simulink model "TRANSMISION_MULTIPLEXADA60EB2"  (R2016a)
settings: Solver=VariableStepAuto  StartTime=0.0  StopTime=420800  RelTol=1e-3
libraries: commutil2 x14, commdigbbndpm3 x14, commsrccod2 x6, commchan3 x2, commsink2 x1
settings Model: Creator=Glynis  LastModifiedBy=Glynis

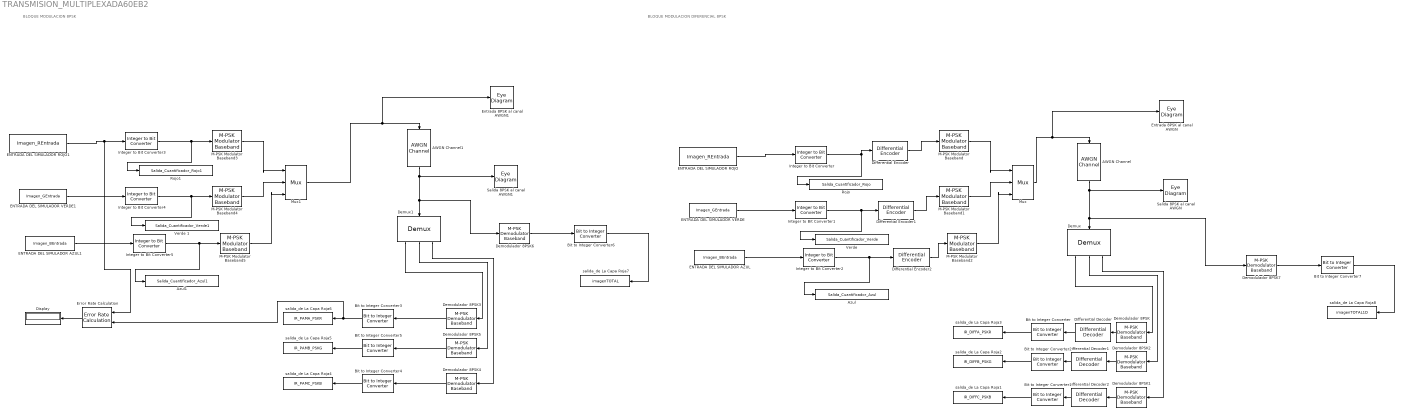
== system TRANSMISION_MULTIPLEXADA60EB2 ==
  note: BLOQUE MODULACION DIFERENCIAL 8PSK
  note: BLOQUE MODULACION 8PSK
  AWGN Channel : commchan3/AWGN Channel  InputProcessing=Columns as channels (frame based)  seed=654  noiseMode="Signal to noise ratio  (Eb/No)"  EbNodB=60  EsNodB=10  SNRdB=10  bitsPerSym=8  Ps=1000  Tsym=1  variance=1
  AWGN Channel1 : commchan3/AWGN Channel  InputProcessing=Columns as channels (frame based)  seed=654  noiseMode="Signal to noise ratio  (Eb/No)"  EbNodB=60  EsNodB=10  SNRdB=10  bitsPerSym=8  Ps=1000  Tsym=1  variance=1
  Azul : ToWorkspace  VariableName=Salida_Cuantificador_Azul  SampleTime=-1
      settings: Save2DSignal=2-D array (concatenate along first dimension)
  Azul1 : ToWorkspace  VariableName=Salida_Cuantificador_Azul1  SampleTime=-1
      settings: Save2DSignal=2-D array (concatenate along first dimension)
  Bit to Integer Converter{,1..7} (8 alike) : commutil2/Bit to Integer Converter  nbits=8  bitOrder=MSB first  signedOutputValues=Unsigned  outDtype=double  outDtypeSigned=Inherit via internal rule
  Demodulador 8PSK{,1..7} (8 alike) : commdigbbndpm3/M-PSK Demodulator Baseband  M=8  OutType=Integer  DecType=Hard decision  VarSource=Dialog  Variance=1  Dec=Gray  Mapping=[0:7]  Ph=pi/8  outDtype1=Inherit via internal rule  outDtype2=Inherit via internal rule  derotateFactorWordLen=16  derotateFactorDataTypeStr=Inherit: Same word length as input  derotateFactorLastDataTypeStr=Inherit: Same word length as input
  Demux : Demux  Outputs=3
  Demux1 : Demux  Outputs=3
  Differential Decoder : commsrccod2/Differential Decoder  InitCond=0
  Differential Decoder1 : commsrccod2/Differential Decoder  InitCond=0
  Differential Decoder2 : commsrccod2/Differential Decoder  InitCond=0
  Differential Encoder : commsrccod2/Differential Encoder  InitCond=0
  Differential Encoder1 : commsrccod2/Differential Encoder  InitCond=0
  Differential Encoder2 : commsrccod2/Differential Encoder  InitCond=0
  Display : Display
  ENTRADA DEL SIMULADOR AZUL : FromWorkspace  VariableName=Imagen_BEntrada  SampleTime=1  OutputAfterFinalValue=Holding final value
  ENTRADA DEL SIMULADOR AZUL1 : FromWorkspace  VariableName=Imagen_BEntrada  SampleTime=1  OutputAfterFinalValue=Holding final value
  ENTRADA DEL SIMULADOR ROJO : FromWorkspace  VariableName=Imagen_REntrada  SampleTime=1  OutputAfterFinalValue=Holding final value
  ENTRADA DEL SIMULADOR ROJO1 : FromWorkspace  VariableName=Imagen_REntrada  SampleTime=1  OutputAfterFinalValue=Holding final value
  ENTRADA DEL SIMULADOR VERDE : FromWorkspace  VariableName=Imagen_GEntrada  SampleTime=1  OutputAfterFinalValue=Holding final value
  ENTRADA DEL SIMULADOR VERDE1 : FromWorkspace  VariableName=Imagen_GEntrada  SampleTime=1  OutputAfterFinalValue=Holding final value
  Entrada 8PSK al canal AWGN : EyeDiagram
  Entrada 8PSK al canal AWGN1 : EyeDiagram
  Error Rate Calculation : commsink2/Error Rate Calculation  N=0  st_delay=0  cp_mode=Entire frame  subframe=[]  PMode=Port  WsName=ErrorVec  RsMode2=off  stop=off  numErr=100  maxBits=1e6
  Integer to Bit Converter{,1..5} (6 alike) : commutil2/Integer to Bit Converter  nbits=8  signedInputValues=Unsigned  bitOrder=MSB first  outDtype=double
  M-PSK Modulator Baseband{,1..5} (6 alike) : commdigbbndpm3/M-PSK Modulator Baseband  M=8  InType=Integer  Enc=Gray  Mapping=[0:7]  Ph=pi/8  outDtype=double  outWordLen=16  outUDDataType=sfix(16)  outFracLenMode=Best precision  outFracLen=15  outDataTypeStr=double  outLastDataTypeStr=double
  Mux : Mux  Inputs=3
      settings: DisplayOption=signals
  Mux1 : Mux  Inputs=3
      settings: DisplayOption=signals
  Rojo : ToWorkspace  VariableName=Salida_Cuantificador_Rojo  SampleTime=-1
      settings: Save2DSignal=2-D array (concatenate along first dimension)
  Rojo1 : ToWorkspace  VariableName=Salida_Cuantificador_Rojo1  SampleTime=-1
      settings: Save2DSignal=2-D array (concatenate along first dimension)
  Salida 8PSK al canal AWGN : EyeDiagram
  Salida 8PSK al canal AWGN1 : EyeDiagram
  "Verde " : ToWorkspace  VariableName=Salida_Cuantificador_Verde  SampleTime=-1
      settings: Save2DSignal=2-D array (concatenate along first dimension)
  Verde 1 : ToWorkspace  VariableName=Salida_Cuantificador_Verde1  SampleTime=-1
      settings: Save2DSignal=2-D array (concatenate along first dimension)
  salida_de La Capa Roja1 : ToWorkspace  VariableName=IR_DIFFC_PSKB  SampleTime=1
      settings: Save2DSignal=2-D array (concatenate along first dimension)
  salida_de La Capa Roja2 : ToWorkspace  VariableName=IR_DIFFB_PSKG  SampleTime=1
      settings: Save2DSignal=2-D array (concatenate along first dimension)
  salida_de La Capa Roja3 : ToWorkspace  VariableName=IR_DIFFA_PSKR  SampleTime=1
      settings: Save2DSignal=2-D array (concatenate along first dimension)
  salida_de La Capa Roja4 : ToWorkspace  VariableName=IR_PAMC_PSKB  SampleTime=1
      settings: Save2DSignal=2-D array (concatenate along first dimension)
  salida_de La Capa Roja5 : ToWorkspace  VariableName=IR_PAMB_PSKG  SampleTime=1
      settings: Save2DSignal=2-D array (concatenate along first dimension)
  salida_de La Capa Roja6 : ToWorkspace  VariableName=IR_PAMA_PSKR  SampleTime=1
      settings: Save2DSignal=2-D array (concatenate along first dimension)
  salida_de La Capa Roja7 : ToWorkspace  VariableName=imagenTOTAL  SampleTime=1
      settings: Save2DSignal=2-D array (concatenate along first dimension)
  salida_de La Capa Roja8 : ToWorkspace  VariableName=imagenTOTAL1D  SampleTime=1
      settings: Save2DSignal=2-D array (concatenate along first dimension)
  wires:
  Integer to Bit Converter/1 -> Rojo/1, Differential Encoder/1
  Bit to Integer Converter/1 -> salida_de La Capa Roja3/1
  ENTRADA DEL SIMULADOR ROJO/1 -> Integer to Bit Converter/1
  Mux/1 -> Entrada 8PSK al canal AWGN/1, AWGN Channel/1
  Demux/1 -> Demodulador 8PSK/1
  Bit to Integer Converter1/1 -> salida_de La Capa Roja1/1
  Bit to Integer Converter2/1 -> salida_de La Capa Roja2/1
  Demux/2 -> Demodulador 8PSK2/1
  Demux/3 -> Demodulador 8PSK1/1
  M-PSK Modulator Baseband/1 -> Mux/1
  Integer to Bit Converter1/1 -> Differential Encoder1/1, "Verde "/1
  ENTRADA DEL SIMULADOR VERDE/1 -> Integer to Bit Converter1/1
  M-PSK Modulator Baseband1/1 -> Mux/2
  Integer to Bit Converter2/1 -> Differential Encoder2/1, Azul/1
  ENTRADA DEL SIMULADOR AZUL/1 -> Integer to Bit Converter2/1
  M-PSK Modulator Baseband2/1 -> Mux/3
  Demodulador 8PSK/1 -> Differential Decoder/1
  Differential Decoder/1 -> Bit to Integer Converter/1
  Differential Decoder1/1 -> Bit to Integer Converter2/1
  Demodulador 8PSK2/1 -> Differential Decoder1/1
  Differential Decoder2/1 -> Bit to Integer Converter1/1
  Demodulador 8PSK1/1 -> Differential Decoder2/1
  Differential Encoder/1 -> M-PSK Modulator Baseband/1
  Differential Encoder1/1 -> M-PSK Modulator Baseband1/1
  Differential Encoder2/1 -> M-PSK Modulator Baseband2/1
  Integer to Bit Converter3/1 -> M-PSK Modulator Baseband3/1, Rojo1/1
  Bit to Integer Converter3/1 -> Error Rate Calculation/2, salida_de La Capa Roja6/1
  ENTRADA DEL SIMULADOR ROJO1/1 -> Error Rate Calculation/1, Integer to Bit Converter3/1
  Demodulador 8PSK3/1 -> Bit to Integer Converter3/1
  Mux1/1 -> Entrada 8PSK al canal AWGN1/1, AWGN Channel1/1
  Demux1/1 -> Demodulador 8PSK3/1
  Bit to Integer Converter4/1 -> salida_de La Capa Roja4/1
  Demodulador 8PSK4/1 -> Bit to Integer Converter4/1
  Bit to Integer Converter5/1 -> salida_de La Capa Roja5/1
  Demodulador 8PSK5/1 -> Bit to Integer Converter5/1
  Demux1/2 -> Demodulador 8PSK5/1
  Demux1/3 -> Demodulador 8PSK4/1
  M-PSK Modulator Baseband3/1 -> Mux1/1
  Integer to Bit Converter4/1 -> M-PSK Modulator Baseband4/1, Verde 1/1
  ENTRADA DEL SIMULADOR VERDE1/1 -> Integer to Bit Converter4/1
  M-PSK Modulator Baseband4/1 -> Mux1/2
  Integer to Bit Converter5/1 -> M-PSK Modulator Baseband5/1, Azul1/1
  ENTRADA DEL SIMULADOR AZUL1/1 -> Integer to Bit Converter5/1
  M-PSK Modulator Baseband5/1 -> Mux1/3
  Error Rate Calculation/1 -> Display/1
  Demodulador 8PSK6/1 -> Bit to Integer Converter6/1
  AWGN Channel1/1 -> Demodulador 8PSK6/1, Demux1/1, Salida 8PSK al canal AWGN1/1
  Bit to Integer Converter6/1 -> salida_de La Capa Roja7/1
  Demodulador 8PSK7/1 -> Bit to Integer Converter7/1
  AWGN Channel/1 -> Demodulador 8PSK7/1, Demux/1, Salida 8PSK al canal AWGN/1
  Bit to Integer Converter7/1 -> salida_de La Capa Roja8/1
